simulink model "LFRefMdl"  (R2023b)
settings: Solver=FixedStepDiscrete  StartTime=0.0  StopTime=inf  FixedStep=Ts  RelTol=1e-3
undefined symbols (not defined in the file or in its folder): Cf, Cr, DataType, default_spacing, hasLag, Iz, lf, lr, m, max_ac, max_steer, min_ac, min_steer, NumEgoStates, posSelector, PredictionHorizon, tau, time_gap, Ts, v0_ego
libraries: mpcsigdimcheck_private x19, mpclib x7, simulink x2, mpcadaslib x1, trackingutilitieslib x1, drivinglib x1
(part 2 of 2)

== system LFRefMdl/MPC Controller /Path Following Control System/MPC Models/MPC Model ==
  Sample time : Inport
  Transport lag : Inport  Port=2
  Longitudinal velocity : Inport  Port=3
  Ag : Inport  Port=4
  Bg : Inport  Port=5
  Cg : Inport  Port=6
  Adaptive Model : MATLAB Function  TreatAsAtomicUnit=on
  Bus Creator2 : BusCreator  Inputs=8
  DX Constant : Constant  Value=zeros(NumEgoStates+2+3*hasLag,1)  VectorParams1D=off  OutDataTypeStr=DataType
  U Constant : Constant  Value=zeros(3,1)  VectorParams1D=off  OutDataTypeStr=DataType
  X Constant : Constant  Value=zeros(NumEgoStates+2+3*hasLag,1)  VectorParams1D=off  OutDataTypeStr=DataType
  Y Constant : Constant  Value=[InitialLongVel;0;0]  VectorParams1D=off  OutDataTypeStr=DataType
  Model : Outport  VectorParamsAs1DForOutWhenUnconnected=off
  wires:
  Cg/1 -> Adaptive Model/5(Cg)
  Bg/1 -> Adaptive Model/4(Bg)
  Ag/1 -> Adaptive Model/3(Ag)
  Bus Creator2/1 -> Model/1
  X Constant/1 -> Bus Creator2/7  "X"
  Y Constant/1 -> Bus Creator2/6  "Y"
  Sample time/1 -> Adaptive Model/1(Ts)
  Adaptive Model/1(A) -> Bus Creator2/1  "A"
  Longitudinal velocity/1 -> Adaptive Model/2(Vx)
  Adaptive Model/4(D) -> Bus Creator2/4  "D"
  Adaptive Model/3(C) -> Bus Creator2/3  "C"
  DX Constant/1 -> Bus Creator2/8  "DX"
  U Constant/1 -> Bus Creator2/5  "U"
  Transport lag/1 -> Adaptive Model/6(lag)
  Adaptive Model/2(B) -> Bus Creator2/2  "B"

== system LFRefMdl/MPC Controller /Path Following Control System/MPC Models/MPC Model with Spacing Control ==
  Sample time : Inport
  Transport lag : Inport  Port=2
  Longitudinal velocity : Inport  Port=3
  Ag : Inport  Port=4
  Bg : Inport  Port=5
  Cg : Inport  Port=6
  Adaptive Model with Spacing Control : MATLAB Function  TreatAsAtomicUnit=on
  Bus Creator2 : BusCreator  Inputs=8
  DX Constant : Constant  Value=zeros(NumEgoStates+3+4*hasLag,1)  VectorParams1D=off  OutDataTypeStr=DataType
  U Constant : Constant  Value=[0;0;InitialLongVel;0]  VectorParams1D=off  OutDataTypeStr=DataType
  X Constant : Constant  Value=zeros(NumEgoStates+3+4*hasLag,1)  VectorParams1D=off  OutDataTypeStr=DataType
  Y Constant : Constant  Value=[1.4*InitialLongVel+DefaultSpacing;InitialLongVel;0;0]  VectorParams1D=off  OutDataTypeStr=DataType
  Model : Outport  VectorParamsAs1DForOutWhenUnconnected=off
  wires:
  Transport lag/1 -> Adaptive Model with Spacing Control/6(lag)
  Cg/1 -> Adaptive Model with Spacing Control/5(Cg)
  Bg/1 -> Adaptive Model with Spacing Control/4(Bg)
  Ag/1 -> Adaptive Model with Spacing Control/3(Ag)
  U Constant/1 -> Bus Creator2/5  "U"
  Y Constant/1 -> Bus Creator2/6  "Y"
  Longitudinal velocity/1 -> Adaptive Model with Spacing Control/2(Vx)
  Adaptive Model with Spacing Control/3(C) -> Bus Creator2/3  "C"
  Adaptive Model with Spacing Control/2(B) -> Bus Creator2/2  "B"
  DX Constant/1 -> Bus Creator2/8  "DX"
  Adaptive Model with Spacing Control/1(A) -> Bus Creator2/1  "A"
  Sample time/1 -> Adaptive Model with Spacing Control/1(Ts)
  Bus Creator2/1 -> Model/1
  X Constant/1 -> Bus Creator2/7  "X"
  Adaptive Model with Spacing Control/4(D) -> Bus Creator2/4  "D"

== system LFRefMdl/MPC Controller /Path Following Control System/Vehicle Models/Vehicle external model ==
  Vehicle dynamics matrix A : Inport
  Vehicle dynamics matrix B : Inport  Port=2
  Vehicle dynamics matrix C : Inport  Port=3
  DataTypeConversion_A : mpcsigdimcheck_private/DataTypeAutoConversion2D  datatypestr=DataType
  DataTypeConversion_B : mpcsigdimcheck_private/DataTypeAutoConversion2D  datatypestr=DataType
  DataTypeConversion_C : mpcsigdimcheck_private/DataTypeAutoConversion2D  datatypestr=DataType
  Signal Specification A : SignalSpecification
  Signal Specification B : SignalSpecification
  Signal Specification C : SignalSpecification
  A : Outport  VectorParamsAs1DForOutWhenUnconnected=off
  B : Outport  Port=2  VectorParamsAs1DForOutWhenUnconnected=off
  C : Outport  Port=3  VectorParamsAs1DForOutWhenUnconnected=off
  wires:
  DataTypeConversion_B/1 -> Signal Specification B/1
  Vehicle dynamics matrix B/1 -> DataTypeConversion_B/1
  DataTypeConversion_A/1 -> Signal Specification A/1
  Vehicle dynamics matrix C/1 -> DataTypeConversion_C/1
  Vehicle dynamics matrix A/1 -> DataTypeConversion_A/1
  Signal Specification A/1 -> A/1
  DataTypeConversion_C/1 -> Signal Specification C/1
  Signal Specification C/1 -> C/1
  Signal Specification B/1 -> B/1

== system LFRefMdl/MPC Controller /Path Following Control System/Vehicle Models/Vehicle parametric model ==
  Vx : Inport
  Vehicle combined dynamics : Subsystem
  Vehicle lateral dynamics : Subsystem
  Vehicle longitudinal dynamics : Subsystem
  A : Outport  VectorParamsAs1DForOutWhenUnconnected=off
  B : Outport  Port=2  VectorParamsAs1DForOutWhenUnconnected=off
  C : Outport  Port=3  VectorParamsAs1DForOutWhenUnconnected=off
  wires:
  Vx/1 -> Vehicle lateral dynamics/1(Vx)
  Vehicle longitudinal dynamics/3(Cn) -> Vehicle combined dynamics/3(C1)
  Vehicle longitudinal dynamics/2(Bn) -> Vehicle combined dynamics/2(B1)
  Vehicle longitudinal dynamics/1(An) -> Vehicle combined dynamics/1(A1)
  Vehicle lateral dynamics/3(Cm) -> Vehicle combined dynamics/6(C2)
  Vehicle lateral dynamics/2(Bm) -> Vehicle combined dynamics/5(B2)
  Vehicle lateral dynamics/1(Am) -> Vehicle combined dynamics/4(A2)
  Vehicle combined dynamics/2(B) -> B/1
  Vehicle combined dynamics/1(A) -> A/1
  Vehicle combined dynamics/3(C) -> C/1

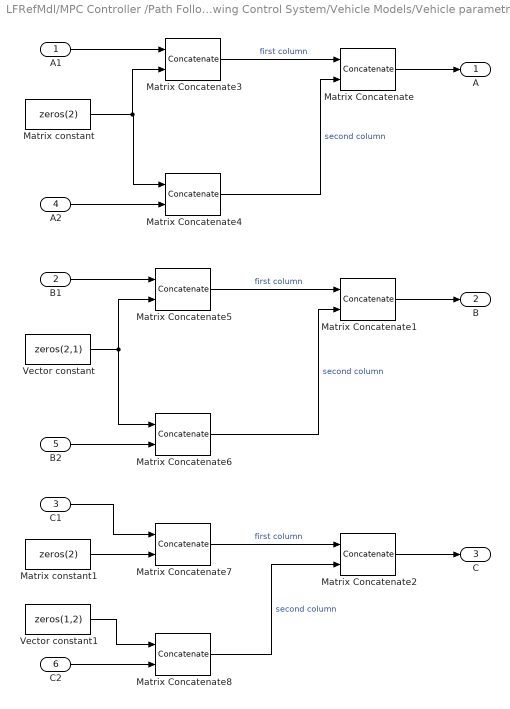
== system LFRefMdl/MPC Controller /Path Following Control System/Vehicle Models/Vehicle parametric model/Vehicle combined dynamics ==
  A1 : Inport
  B1 : Inport  Port=2
  C1 : Inport  Port=3
  A2 : Inport  Port=4
  B2 : Inport  Port=5
  C2 : Inport  Port=6
  Matrix Concatenate : Concatenate  Mode=Multidimensional array  ConcatenateDimension=2
  Matrix Concatenate1 : Concatenate  Mode=Multidimensional array  ConcatenateDimension=2
  Matrix Concatenate2 : Concatenate  Mode=Multidimensional array  ConcatenateDimension=2
  Matrix Concatenate{3..8} (6 alike) : Concatenate  Mode=Multidimensional array
  Matrix constant : Constant  Value=zeros(2)  VectorParams1D=off  OutDataTypeStr=DataType
  Matrix constant1 : Constant  Value=zeros(2)  VectorParams1D=off  OutDataTypeStr=DataType
  Vector constant : Constant  Value=zeros(2,1)  VectorParams1D=off  OutDataTypeStr=DataType
  Vector constant1 : Constant  Value=zeros(1,2)  VectorParams1D=off  OutDataTypeStr=DataType
  A : Outport  VectorParamsAs1DForOutWhenUnconnected=off
  B : Outport  Port=2  VectorParamsAs1DForOutWhenUnconnected=off
  C : Outport  Port=3  VectorParamsAs1DForOutWhenUnconnected=off
  wires:
  Matrix Concatenate5/1 -> Matrix Concatenate1/1  "first column"
  A1/1 -> Matrix Concatenate3/1
  Matrix Concatenate3/1 -> Matrix Concatenate/1  "first column"
  A2/1 -> Matrix Concatenate4/2
  B2/1 -> Matrix Concatenate6/2
  C2/1 -> Matrix Concatenate8/2
  Matrix Concatenate7/1 -> Matrix Concatenate2/1  "first column"
  Matrix Concatenate8/1 -> Matrix Concatenate2/2  "second column"
  Matrix constant1/1 -> Matrix Concatenate7/2
  Matrix Concatenate2/1 -> C/1
  Matrix constant/1 -> Matrix Concatenate3/2, Matrix Concatenate4/1
  Matrix Concatenate/1 -> A/1
  Vector constant1/1 -> Matrix Concatenate8/1
  Matrix Concatenate1/1 -> B/1
  B1/1 -> Matrix Concatenate5/1
  Matrix Concatenate4/1 -> Matrix Concatenate/2  "second column"
  Matrix Concatenate6/1 -> Matrix Concatenate1/2  "second column"
  C1/1 -> Matrix Concatenate7/1
  Vector constant/1 -> Matrix Concatenate5/2, Matrix Concatenate6/1

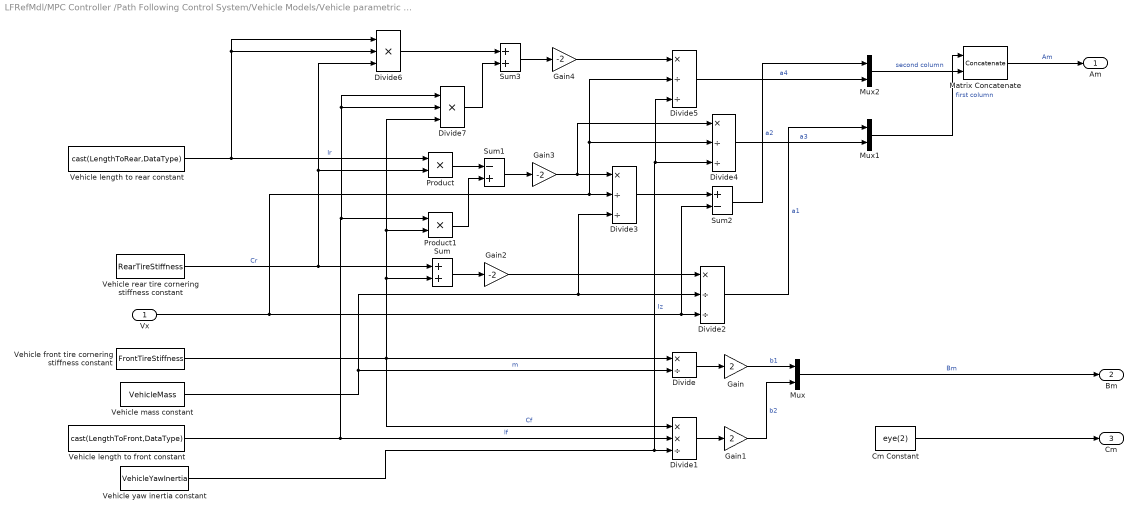
== system LFRefMdl/MPC Controller /Path Following Control System/Vehicle Models/Vehicle parametric model/Vehicle lateral dynamics ==
  Vx : Inport
  Cm Constant : Constant  Value=eye(2)  OutDataTypeStr=DataType
  Divide : Product  Inputs=*/
  Divide1 : Product  Inputs=**/
  Divide{2..5} (4 alike) : Product  Inputs=*//
  Divide6 : Product  Inputs=***
  Divide7 : Product  Inputs=***
  Gain : Gain  Gain=2
  Gain1 : Gain  Gain=2
  Gain2 : Gain  Gain=-2
  Gain3 : Gain  Gain=-2
  Gain4 : Gain  Gain=-2
  Matrix Concatenate : Concatenate  Mode=Multidimensional array  ConcatenateDimension=2
  Mux : Mux  Inputs=[1 1]
  Mux1 : Mux  Inputs=[1 1]
  Mux2 : Mux  Inputs=[1 1]
  Product : Product
  Product1 : Product
  Sum : Sum
  Sum1 : Sum  Inputs=-+
  Sum2 : Sum  Inputs=+-
  Sum3 : Sum
  Vehicle front tire cornering stiffness constant : Constant  Value=FrontTireStiffness  OutDataTypeStr=DataType
  Vehicle length to front constant : Constant  Value=cast(LengthToFront,DataType)  OutDataTypeStr=DataType
  Vehicle length to rear constant : Constant  Value=cast(LengthToRear,DataType)  OutDataTypeStr=DataType
  Vehicle mass constant : Constant  Value=VehicleMass  OutDataTypeStr=DataType
  Vehicle rear tire cornering stiffness constant : Constant  Value=RearTireStiffness  OutDataTypeStr=DataType
  Vehicle yaw inertia constant : Constant  Value=VehicleYawInertia  OutDataTypeStr=DataType
  Am : Outport  VectorParamsAs1DForOutWhenUnconnected=off
  Bm : Outport  Port=2  VectorParamsAs1DForOutWhenUnconnected=off
  Cm : Outport  Port=3  VectorParamsAs1DForOutWhenUnconnected=off
  wires:
  Divide6/1 -> Sum3/1
  Gain2/1 -> Divide2/1
  Cm Constant/1 -> Cm/1
  Divide1/1 -> Gain1/1
  Divide/1 -> Gain/1
  Gain1/1 -> Mux/2  "b2"
  Divide3/1 -> Sum2/1
  Sum/1 -> Gain2/1
  Mux1/1 -> Matrix Concatenate/1  "first column"
  Sum1/1 -> Gain3/1
  Gain3/1 -> Divide4/1, Divide3/1
  Sum3/1 -> Gain4/1
  Matrix Concatenate/1 -> Am/1  "Am"
  Divide7/1 -> Sum3/2
  Divide4/1 -> Mux1/2  "a3"
  Mux/1 -> Bm/1  "Bm"
  Product/1 -> Sum1/1
  Divide2/1 -> Mux1/1  "a1"
  Gain/1 -> Mux/1  "b1"
  Vx/1 -> Divide2/3, Sum2/2, Divide4/2, Divide5/2, Divide3/2
  Sum2/1 -> Mux2/1  "a2"
  Vehicle rear tire cornering stiffness constant/1 -> Sum/1, Product/2, Divide6/3  "Cr"
  Vehicle length to rear constant/1 -> Product/1, Divide6/1, Divide6/2  "lr"
  Gain4/1 -> Divide5/1
  Vehicle mass constant/1 -> Divide2/2, Divide3/3, Divide/2  "m"
  Vehicle yaw inertia constant/1 -> Divide1/3, Divide4/3, Divide5/3  "Iz"
  Vehicle front tire cornering stiffness constant/1 -> Sum/2, Product1/2, Divide7/3, Divide/1, Divide1/1  "Cf"
  Product1/1 -> Sum1/2
  Mux2/1 -> Matrix Concatenate/2  "second column"
  Vehicle length to front constant/1 -> Divide1/2, Product1/1, Divide7/2, Divide7/1  "lf"
  Divide5/1 -> Mux2/2  "a4"

== system LFRefMdl/MPC Controller /Path Following Control System/Vehicle Models/Vehicle parametric model/Vehicle longitudinal dynamics ==
  Cn constant : Constant  Value=[0,1]  VectorParams1D=off  OutDataTypeStr=DataType
  Divide : Product  Inputs=*/
  Matrix Concatenate : Concatenate  Mode=Multidimensional array  ConcatenateDimension=2
  Mux1 : Mux  Inputs=[1 1]
  Mux2 : Mux  Inputs=[1 1]
  Scalar one constant : Constant  OutDataTypeStr=DataType
  Scalar zero constant : Constant  Value=0  OutDataTypeStr=DataType
  Unary Minus : UnaryMinus
  Vector constant : Constant  Value=zeros(2,1)  VectorParams1D=off  OutDataTypeStr=DataType
  Vehicle acceleration tracking time constant : Constant  Value=AccelTimeConstant  OutDataTypeStr=DataType
  An : Outport  VectorParamsAs1DForOutWhenUnconnected=off
  Bn : Outport  Port=2  VectorParamsAs1DForOutWhenUnconnected=off
  Cn : Outport  Port=3  VectorParamsAs1DForOutWhenUnconnected=off
  wires:
  Mux1/1 -> Matrix Concatenate/1  "first column"
  Scalar zero constant/1 -> Mux2/2
  Mux2/1 -> Bn/1  "Bn"
  Scalar one constant/1 -> Divide/1, Mux1/2  "a3"
  Unary Minus/1 -> Mux1/1  "a1"
  Cn constant/1 -> Cn/1  "Cn"
  Matrix Concatenate/1 -> An/1  "An"
  Vector constant/1 -> Matrix Concatenate/2  "second column"
  Divide/1 -> Unary Minus/1, Mux2/1  "1/tau"
  Vehicle acceleration tracking time constant/1 -> Divide/2  "tau"

== stateflow chart LFRefMdl/Test Assessment ==
  state Scenario_1
    state Assessments
      state CheckFirst
        verify(lateral_deviation<10 && lateral_deviation>-10)
      state else
      (default) -> (junction 174)
      Assessments -> (junction 174)
      (junction 174) -> (junction 175) [order 1] : [true
          | ]
      (junction 175) -> CheckFirst [order 1] : [~in(Scenario_1.Assessments.CheckFirst)]
      (junction 174) -> (junction 183) [order 2]
      (junction 175) -> (junction 178) [order 2]
      (junction 183) -> (junction 184)
      (junction 184) -> else [order 1] : [~in(Scenario_1.Assessments.else)]
      (junction 184) -> (junction 187) [order 2]
    (default) -> Assessments
  (default) -> Scenario_1 : {assert(Active_Scenario_Index == 1,'The value of Scenario Parameter ''Active_Scenario_Index'' is not valid. Use the index of the scenario to specify it.')}
  data: lateral_deviation input; Active_Scenario_Index parameter =1

== stateflow chart LFRefMdl/Test Sequence ==
  state Scenario_1
    state step_1
      set_velocity = Driver_Set_Velocity;
    (default) -> step_1
  (default) -> Scenario_1 : {assert(Active_Scenario_Index == 1,'The value of Scenario Parameter ''Active_Scenario_Index'' is not valid. Use the index of the scenario to specify it.')}
  data: Driver_Set_Velocity input; set_velocity output; Active_Scenario_Index parameter =1

== stateflow chart LFRefMdl/FitnessConverter_Hecate ==
  state Assessments
    fitness_1 = Inf;
    state CheckFirst
      fitness_1 = min([10-(lateral_deviation);lateral_deviation-(-10);]);
    state else
      fitness_1 = Inf;
    (default) -> (junction 4)
    else -> (junction 4) : [(true)]
    (junction 4) -> CheckFirst [order 1] : [true]
    (junction 4) -> else [order 2] : []
    CheckFirst -> (junction 4) : [~(true)]
  (default) -> Assessments
  data: lateral_deviation input; fitness_1 output

== matlab function LFRefMdl/Tracking and Sensor Fusion/Find Lead Car ==
  data: confirmedTracks input; x output size=[1 1]; vx output size=[1 1]; lane input; mioTrackIndex output; positionSelector input
function [x,vx,mioTrackIndex] = findLeadCar(confirmedTracks, lane, positionSelector)
% This function finds the lead car: a car in front of the ego car that
% satisfies all the criteria below:
% * Within the ego car's lane.
% * In front of the ego car.
% * Closest to the ego car.

% Note: If you change state definition, change the following:
%       State = [x;vx;y;vy;z;vz] (3D constant velocity)
numStates = 6;

% Initialize outputs and parameters
maxX = cast(1000, 'like', confirmedTracks.Tracks(1).State);  % Far enough forward so that no track is expected to exceed this distance
mioTrackIndex = 0;

% If lane detection is not available, the ego car is assumed to be located
% in the middle of its lane. The lane width is assumed to be 3.6m, typical
% highway lane width.
laneWidth = 3.6;
halfLaneWidth = laneWidth/2;

if lane.Left.Strength > 0.01
    lb = [lane.Left.CurvatureDerivative/6,...
        lane.Left.Curvature/2,...
        lane.Left.HeadingAngle,...
        lane.Left.LateralOffset];
else
    lb = single([0,0,0,halfLaneWidth]);
end

if lane.Right.Strength > 0.01
    rb = [lane.Right.CurvatureDerivative/6,...
        lane.Right.Curvature/2,...
        lane.Right.HeadingAngle,...
        lane.Right.LateralOffset];
else
    rb = single([0,0,0,-halfLaneWidth]);    
end

for i = 1:confirmedTracks.NumTracks
    position = positionSelector * confirmedTracks.Tracks(i).State;
    x = position(1); % Longitudinal position of the track relative to ego
    y = position(2); % Lateral position of the track relative to ego
    
    if x < maxX && x > 0 % No point checking otherwise

        yleftLane  = polyval(lb,x); % lateral position of left lane
        yrightLane = polyval(rb,x); % lateral position of right lane
        
        % Find a new lead car
        if (yrightLane <= y) && (y <= yleftLane)
            maxX = x;
            mioTrackIndex(:) = i;
        end
    end
end

if mioTrackIndex>0
    mioState = confirmedTracks.Tracks(mioTrackIndex).State;
else
    mioState = inf(numStates,1,'like',confirmedTracks.Tracks(1).State);
end

% Output:
x = mioState(1);    % Longitudinal position of the lead car
vx = mioState(2);   % Longitudinal velocity of the lead car

== matlab function LFRefMdl/MPC Controller /Path Following Control System/MPC Models/MPC Model/Adaptive Model ==
  data: Ts input; A output; Vx input; Ag input; Bg input; Cg input; lag input; B output; C output; D output; hasLag parameter
  function [A,B,C,D] = getAdaptiveMPCModel(Ts,Vx,Ag, Bg, Cg, lag, hasLag)
% Get discrete state-space model for Adaptive MPC with sample time Ts.
% Called by the 'Path Following Control System' Block.

% Inputs:
%   Ts:               mask variable for sample time
%   Vx:               mask inport for longitudinal velocity
%   Ag,Bg,Cg:         continuous or discrete vehicle model with sample time Ts    
%   hasLag:           indicating if lag>0 (true or false)
% Outputs:
%   A,B,C,D:          discrete time model for adaptive MPC

%   Author: Meng Xia, Rong Chen
%   Copyright 2017-2018 The MathWorks, Inc.

% Discrete MPC model
[A,B,C,D] = pfcblock_utilGetDiscreteModelForMPCNoSpacingCtrl(Ts,Vx,Ag,Bg,Cg,lag,hasLag);

== matlab function LFRefMdl/MPC Controller /Path Following Control System/Data Processing for MPC Controller/DataTypeConversion_extmv ==
  data: u input size=[2 1]; y output; isDouble parameter
function y = fcn(u,isDouble)
if isDouble
    if isa(u,'double')
        y = u;
    else
        y = double(u);
    end
else
    if isa(u,'single')
        y = u;
    else
        y = single(u);
    end
end

== matlab function LFRefMdl/MPC Controller /Path Following Control System/MPC Models/MPC Model with Spacing Control/Adaptive Model with Spacing Control ==
  data: Ts input; A output; Vx input; Ag input; Bg input; Cg input; lag input; B output; C output; D output; hasLag parameter
  function [A,B,C,D] = getAdaptiveMPCModel(Ts,Vx,Ag, Bg, Cg, lag,hasLag)
% Get discrete state-space model for Adaptive MPC with sample time Ts.
% Called by the 'Path Following Control System' Block.

% Inputs:
%   Ts:               mask variable for sample time
%   Vx:               mask inport for longitudinal velocity
%   Ag,Bg,Cg:         continuous or discrete vehicle model with sample time Ts       
%   hasLag:           indicating if lag>0 (true or false)
% Outputs:
%   A,B,C,D:          discrete time model for adaptive MPC

%   Author: Meng Xia, Rong Chen
%   Copyright 2017-2018 The MathWorks, Inc.

% Discrete MPC model
[A,B,C,D] = pfcblock_utilGetDiscreteModelForMPCHasSpacingCtrl(Ts,Vx,Ag,Bg,Cg,lag,hasLag);

== matlab function LFRefMdl/Estimate Lane Center/MATLAB Function ==
  data: lanes input
  events: fcnLeftAndRight output FUNCTION_CALL_EVENT; fcnLeftOnly output FUNCTION_CALL_EVENT; fcnRightOnly output FUNCTION_CALL_EVENT; fcnNone output FUNCTION_CALL_EVENT
function fcn(lanes)

leftStrength  = lanes.Left.Strength;
rightStrength = lanes.Right.Strength;

if (leftStrength > 0) && (rightStrength > 0)
   fcnLeftAndRight();
   
elseif leftStrength > 0
    fcnLeftOnly();
    
elseif rightStrength > 0
    fcnRightOnly();
    
else
    fcnNone();
end
